simulink model "PIDControlDMS"  (R2021a)
settings: Solver=FixedStepAuto  StartTime=0.0  StopTime=SimTime-Ts  FixedStep=0.001  RelTol=1e-3
values from neighbouring files (symbols this model uses):
  C12 = x(3)    [DigitalPIDRunner.m]    (also in DoubleMassRunner.m; NNIdentify.m = Xnt_noise(3); NNTrainingSet.m = T(i, 3); PIDModalController.m = 16.6338)
  k1 = x(1)    [DigitalPIDRunner.m]    (also in DoubleMassRunner.m; NNIdentify.m = Xnt_noise(1); NNTrainingSet.m = T(i, 1); PIDModalController.m = 0.2244)
  k2 = x(2)    [DigitalPIDRunner.m]    (also in DoubleMassRunner.m; NNIdentify.m = Xnt_noise(2); NNTrainingSet.m = T(i, 2); PIDModalController.m = 0.5636)
  Kd = 1    [DigitalPIDRunner.m]    (also in PIDModalController.m = (a2j*Omega - a1)/b0; PIDRunner.m = X(3); PolynomialController.m = (a2j*Omega - a1)/b0)
  Ki = 10    [DigitalPIDRunner.m]    (also in PIDModalController.m = (a0j*Omega^3)/b0; PIDRunner.m = X(2); PolynomialController.m = (a0j*Omega^3)/b0)
  Kp = 3    [DigitalPIDRunner.m]    (also in PIDModalController.m = (a1j*Omega^2 - a0)/b0; PIDRunner.m = X(1); PolynomialController.m = (a1j*Omega^2 - a0)/b0)
  Ts = 1e-3    (= 0.001)    [DigitalPIDRunner.m]    (also in DoubleMassRunner.m = ref.Ts; NNTrainingSet.m; PIDModalController.m; PIDRunner.m = p.Results.StepTime)
settings Model: Creator=akangmufti  LastModifiedBy=akangmufti

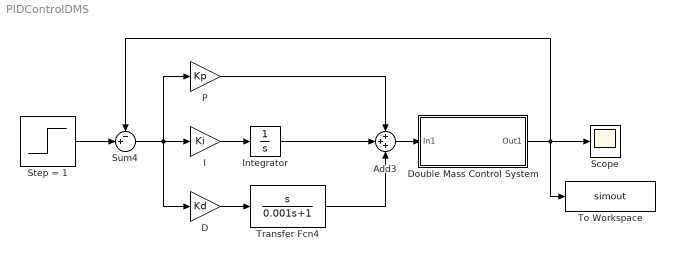
== system PIDControlDMS ==
  Add3 : Sum  Inputs=+++
  D : Gain  Gain=Kd
  Double Mass Control System : Subsystem
  I : Gain  Gain=Ki
  Integrator : Integrator
  P : Gain  Gain=Kp
  Scope : Scope
  Step = 1 : Step  Time=0.0001  SampleTime=0
  Sum4 : Sum  Inputs=-+|
  To Workspace : ToWorkspace  VariableName=simout  SampleTime=Ts
      settings: Save2DSignal=2-D array (concatenate along first dimension)
  Transfer Fcn4 : TransferFcn  Numerator=[1 0]  Denominator=[0.001 1]
  wires:
  Transfer Fcn4/1 -> Add3/3
  Integrator/1 -> Add3/2
  P/1 -> Add3/1
  I/1 -> Integrator/1
  D/1 -> Transfer Fcn4/1
  Step = 1/1 -> Sum4/2
  Sum4/1 -> D/1, P/1, I/1
  Add3/1 -> Double Mass Control System/1(In1)
  Double Mass Control System/1(Out1) -> Sum4/1, To Workspace/1, Scope/1

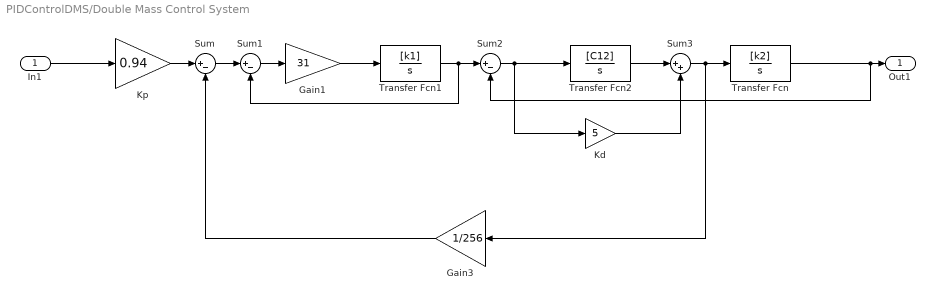
== system PIDControlDMS/Double Mass Control System ==
  In1 : Inport
  Gain1 : Gain  Gain=31
  Gain3 : Gain  Gain=1/256
  Kd : Gain  Gain=5
  Kp : Gain  Gain=0.94
  Sum : Sum  Inputs=|+-
  Sum1 : Sum  Inputs=|+-
  Sum2 : Sum  Inputs=|+-
  Sum3 : Sum  Inputs=|++
  Transfer Fcn : TransferFcn  Numerator=[k2]  Denominator=[1 0]
  Transfer Fcn1 : TransferFcn  Numerator=[k1]  Denominator=[1 0]
  Transfer Fcn2 : TransferFcn  Numerator=[C12]  Denominator=[1 0]
  Out1 : Outport
  wires:
  Kp/1 -> Sum/1
  Transfer Fcn1/1 -> Sum2/1, Sum1/2
  Gain1/1 -> Transfer Fcn1/1
  Sum2/1 -> Kd/1, Transfer Fcn2/1
  Sum1/1 -> Gain1/1
  Gain3/1 -> Sum/2
  Sum/1 -> Sum1/1
  Sum3/1 -> Transfer Fcn/1, Gain3/1
  Transfer Fcn2/1 -> Sum3/1
  In1/1 -> Kp/1
  Kd/1 -> Sum3/2
  Transfer Fcn/1 -> Sum2/2, Out1/1
